simulink model "buttons_to_pwm"  (R2017a)
settings: Solver=VariableStepAuto  StartTime=0.0  StopTime=50000  RelTol=1e-3
libraries: hdlsllib x4, simulink x2
settings Model: Creator=wachala.j  LastModifiedBy=wachala.j

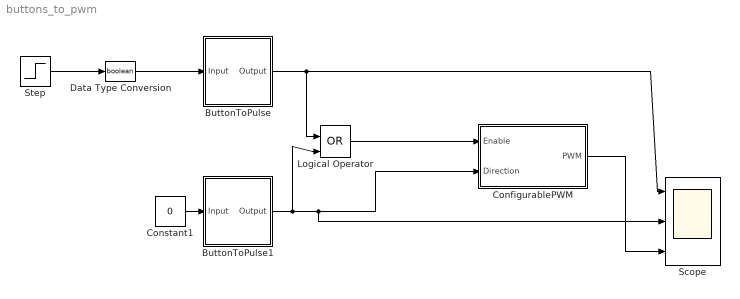
== system buttons_to_pwm ==
  ButtonToPulse : Subsystem
  ButtonToPulse1 : Subsystem
  ConfigurablePWM : Subsystem
  Constant1 : Constant  Value=0  OutDataTypeStr=boolean
  Data Type Conversion : DataTypeConversion  OutDataTypeStr=boolean
  Logical Operator : Logic  Operator=OR  IconShape=distinctive  AllPortsSameDT=off  OutDataTypeStr=boolean
  Scope : Scope  NumInputPorts=3
  Step : Step  Time=25000  Before=1  After=0  SampleTime=1
  wires:
  ButtonToPulse1/1(Output) -> Logical Operator/2, Scope/2, ConfigurablePWM/2(Direction)
  ButtonToPulse/1(Output) -> Scope/1, Logical Operator/1
  Logical Operator/1 -> ConfigurablePWM/1(Enable)
  ConfigurablePWM/1(PWM) -> Scope/3
  Constant1/1 -> ButtonToPulse1/1(Input)
  Step/1 -> Data Type Conversion/1
  Data Type Conversion/1 -> ButtonToPulse/1(Input)

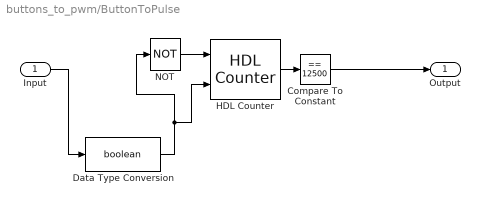
== system buttons_to_pwm/ButtonToPulse ==
  Input : Inport
  Compare To Constant : simulink/Logic and Bit Operations/Compare To Constant  relop===  const=12500  OutDataTypeStr=boolean
  Data Type Conversion : DataTypeConversion  OutDataTypeStr=boolean
  HDL Counter : hdlsllib/HDL Operations/HDL Counter  CountType=Count limited  CountInit=0  CountStep=1  CountMax=50000  CountFromType=Initial value  CountFrom=0  CountResetPort=on  CountLoadPort=off  CountEnbPort=on  CountDirPort=off  CountDataType=Unsigned  CountWordLen=32  CountFracLen=0  CountSampTime=1
      settings: SourceProductName=HDL Coder  SourceProductBaseCode=HD
  NOT : Logic  Operator=NOT  IconShape=distinctive  AllPortsSameDT=off  OutDataTypeStr=boolean
  Output : Outport
  wires:
  NOT/1 -> HDL Counter/1
  Data Type Conversion/1 -> HDL Counter/2, NOT/1
  HDL Counter/1 -> Compare To Constant/1
  Input/1 -> Data Type Conversion/1
  Compare To Constant/1 -> Output/1

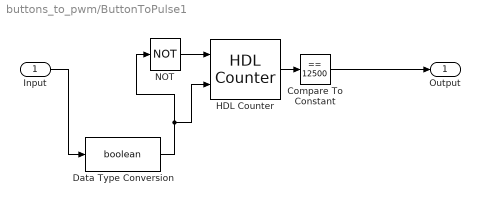
== system buttons_to_pwm/ButtonToPulse1 ==
  Input : Inport
  Compare To Constant : simulink/Logic and Bit Operations/Compare To Constant  relop===  const=12500  OutDataTypeStr=boolean
  Data Type Conversion : DataTypeConversion  OutDataTypeStr=boolean
  HDL Counter : hdlsllib/HDL Operations/HDL Counter  CountType=Count limited  CountInit=0  CountStep=1  CountMax=50000  CountFromType=Initial value  CountFrom=0  CountResetPort=on  CountLoadPort=off  CountEnbPort=on  CountDirPort=off  CountDataType=Unsigned  CountWordLen=32  CountFracLen=0  CountSampTime=1
      settings: SourceProductName=HDL Coder  SourceProductBaseCode=HD
  NOT : Logic  Operator=NOT  IconShape=distinctive  AllPortsSameDT=off  OutDataTypeStr=boolean
  Output : Outport
  wires:
  NOT/1 -> HDL Counter/1
  Data Type Conversion/1 -> HDL Counter/2, NOT/1
  HDL Counter/1 -> Compare To Constant/1
  Input/1 -> Data Type Conversion/1
  Compare To Constant/1 -> Output/1

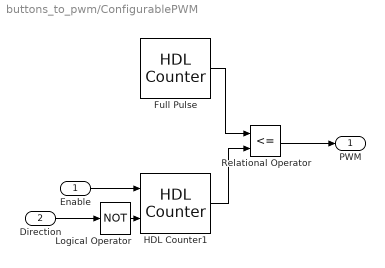
== system buttons_to_pwm/ConfigurablePWM ==
  Enable : Inport  OutDataTypeStr=boolean
  Direction : Inport  Port=2  OutDataTypeStr=boolean
  Full Pulse : hdlsllib/HDL Operations/HDL Counter  CountType=Count limited  CountInit=0  CountStep=1  CountMax=1000  CountFromType=Initial value  CountFrom=0  CountResetPort=off  CountLoadPort=off  CountEnbPort=off  CountDirPort=off  CountDataType=Unsigned  CountWordLen=32  CountFracLen=0  CountSampTime=1
      settings: SourceProductName=HDL Coder  SourceProductBaseCode=HD
  HDL Counter1 : hdlsllib/HDL Operations/HDL Counter  CountType=Count limited  CountInit=30  CountStep=6  CountMax=120  CountFromType=Initial value  CountFrom=30  CountResetPort=off  CountLoadPort=off  CountEnbPort=on  CountDirPort=on  CountDataType=Unsigned  CountWordLen=8  CountFracLen=0  CountSampTime=1
      settings: SourceProductName=HDL Coder  SourceProductBaseCode=HD
  Logical Operator : Logic  Operator=NOT  IconShape=distinctive  AllPortsSameDT=off  OutDataTypeStr=boolean
  Relational Operator : RelationalOperator  Operator=<=  OutDataTypeStr=boolean  RndMeth=Simplest
  PWM : Outport
  wires:
  Relational Operator/1 -> PWM/1
  HDL Counter1/1 -> Relational Operator/2
  Full Pulse/1 -> Relational Operator/1
  Enable/1 -> HDL Counter1/1
  Direction/1 -> Logical Operator/1
  Logical Operator/1 -> HDL Counter1/2
